simulink model "feedforward2"  (R2019b)
settings: Solver=VariableStepAuto  StartTime=0.0  StopTime=1  RelTol=1e-3  EnableMultiTasking=on
undefined symbols (not defined in the file): den4, K2, L2, num4, sigbuilder_block, sysog
settings Model: Creator=zap  LastModifiedBy=bhisma
settings DataIOCC: LimitDataPoints=on  ReturnWorkspaceOutputs=off
settings OptimizationCC: LifeSpan=inf
settings DebuggingCC: AllowSymbolicDim=off  SFUnexpectedBacktrackingDiag=warning  SFNoUnconditionalDefaultTransitionDiag=warning  SFExecutionAtInitializationDiag=none  ArithmeticOperatorsInVariantConditions=warning
settings ModelReferenceCC: PropagateSignalLabelsOutOfModel=off
settings SFSimCC: SimUseLocalCustomCode=off  CustomCodeUndefinedFunction=UseInterfaceOnly
settings RTWCC: RTWUseLocalCustomCode=off
settings CodeAppCC: StateflowObjectComments=on
settings GRTTargetCC: TargetLangStandard=C89/C90 (ANSI)
settings ConfigComp: CovMetricSettings=dw  CovHtmlReporting=on  CovSaveCumulativeToWorkspaceVar=on  CovSaveSingleToWorkspaceVar=on  CovExternalEMLEnable=off

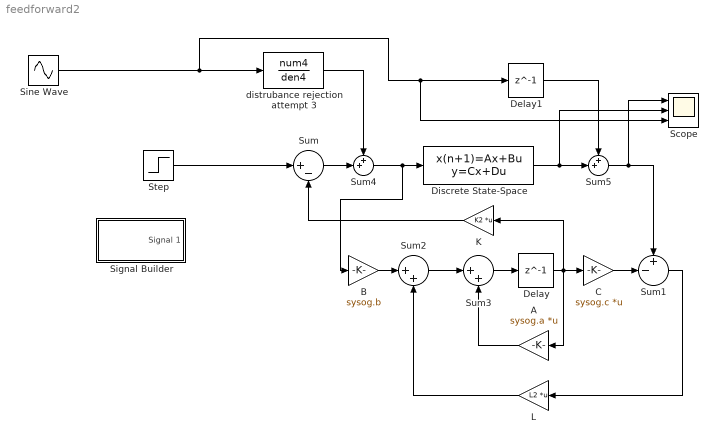
== system feedforward2 ==
  A : Gain  Gain=sysog.a  Multiplication=Matrix(K*u)
  B : Gain  Gain=sysog.b
  C : Gain  Gain=sysog.c  Multiplication=Matrix(K*u)
  Delay : Delay  DelayLength=1  InitialCondition=0
  Delay1 : Delay  DelayLength=1
  Discrete State-Space : DiscreteStateSpace  A=sysog.a  B=sysog.b  C=sysog.c  D=sysog.d  SampleTime=10^-4
  K : Gain  Gain=K2  Multiplication=Matrix(K*u)
  L : Gain  Gain=L2  Multiplication=Matrix(K*u)
  Scope : Scope  NumInputPorts=3
  Signal Builder : Subsystem  Tag=STV Subsys  LoadFcn=sigbuilder_block('load');  StartFcn=sigbuilder_block('start');  StopFcn=sigbuilder_block('stop');  ClipboardFcn=sigbuilder_block('clipboard');  mask(Sigbuilder block){tuvar=[0:10]}
      mask help: Simulink:masks:SigbuilderBlock_MD
      mask init:
      | if ~strcmp(get_param(bdroot(gcbh),'SimulationStatus'),'stopped') tuvar = sigbuilder_block('maskInit'); end
      settings: CopyFcn=sigbuilder_block('copy');  DeleteFcn=sigbuilder_block('delete');  ModelCloseFcn=sigbuilder_block('modelClose');  PreSaveFcn=sigbuilder_block('preSave');  PauseFcn=sigbuilder_block('pause');  ContinueFcn=sigbuilder_block('continue');  NameChangeFcn=sigbuilder_block('namechange');  OpenFcn=sigbuilder_block('open',[437.25 199.5 550.5 399.75 ]);  CloseFcn=sigbuilder_block('close');
      mask Display: plot(0, 0, 100, 100,[2, 2, 32, 32, 2], [68, 8, 8, 68, 68],[32, 2], [38, 38], [32, 19, 2],[53, 60, 44], [32, 17, 17, 2],[16, 16, 31, 31]);txt = getActiveGroup(gcbh);text(2, 100, txt,'verticalAlignment', 'top');
  Sine Wave : Sin  Amplitude=0.1  Frequency=10  SampleTime=10^(-4)
  Step : Step  Time=0  After=1/57  SampleTime=10^-4
  Sum : Sum  Inputs=|+-
  Sum1 : Sum  Inputs=+-|
  Sum2 : Sum  Inputs=|++
  Sum3 : Sum  Inputs=|++
  Sum4 : Sum  Inputs=++|
  Sum5 : Sum  Inputs=++|
  distrubance rejection attempt 3 : DiscreteTransferFcn  Numerator=num4  Denominator=den4  SampleTime=10^-4
  wires:
  Sum/1 -> Sum4/2
  B/1 -> Sum2/1
  Sum2/1 -> Sum3/1
  Sum3/1 -> Delay/1
  A/1 -> Sum3/2
  Delay/1 -> K/1, C/1, A/1
  C/1 -> Sum1/2
  Sum1/1 -> L/1
  L/1 -> Sum2/2
  K/1 -> Sum/2
  Sum4/1 -> B/1, Discrete State-Space/1
  distrubance rejection attempt 3/1 -> Sum4/1
  Discrete State-Space/1 -> Scope/2, Sum5/2
  Sum5/1 -> Scope/1, Sum1/1
  Delay1/1 -> Sum5/1
  Sine Wave/1 -> Scope/3, Delay1/1, distrubance rejection attempt 3/1
  Step/1 -> Sum/1

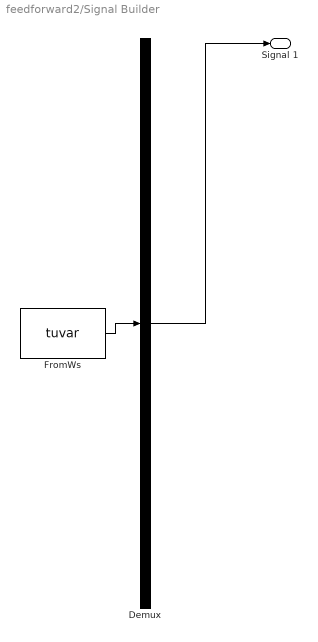
== system feedforward2/Signal Builder ==
  Demux : Demux  Tag=STV Demux  Outputs=1
  FromWs : FromWorkspace  Tag=STV FromWs  VariableName=tuvar  SampleTime=10^(-4)  OutputAfterFinalValue=Holding final value
      SigBuilderData=|
      | common.afterFinalStr = 'Hold final value'
      | common.sampleTime = '10^(-4)'
      | dataSet.timeRange = [0 0.15]
      | dataSet.name = 'Group 1'
      | sbobj.Groups.Name = 'Group 1'
      | sbobj.Groups.Signals.Name = 'Signal 1'
      | sbobj.Groups.Signals.XData = [0 0.025 0.05 0.075 0.1 0.15]
      | sbobj.Groups.Signals.YData = [0 0.0175438596491 0 0.0175438596491 0 0]
      | sbobj.Groups.TimeRange = [0 0.15]
  Signal 1 : Outport  Tag=STV Outport
  wires:
  Demux/1 -> Signal 1/1
  FromWs/1 -> Demux/1
